simulink model "Practica_10_BER_PNRZ"  (R2020a)
settings: Solver=VariableStepAuto  StartTime=0.0  StopTime=StopTime  RelTol=1e-3
libraries: commutil2 x2, commchan3 x1, commrandsrc3 x1, commsink2 x1
settings Model: Creator=León Mora  LastModifiedBy=León Mora

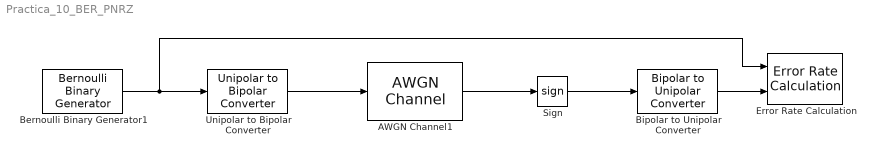
== system Practica_10_BER_PNRZ ==
  AWGN Channel1 : commchan3/AWGN Channel  InputProcessing=Columns as channels (frame based)  seed=67  noiseMode="Signal to noise ratio  (Eb/No)"  EbNodB=EbNo_k  EsNodB=10  SNRdB=10  bitsPerSym=1  Ps=1  Tsym=1  variance=1
  Bernoulli Binary Generator1 : commrandsrc3/Bernoulli Binary Generator  ProbabilityOfZero=0.5  SeedSource=Auto  Seed=0  SampleTime=1  SamplesPerFrame=FrameSize  OutputDataType=double  SimulateUsing=Interpreted execution
  Bipolar to Unipolar Converter : commutil2/Bipolar to Unipolar Converter  M=2  polarity=Positive  dataType=Inherit via internal rule
      settings: SourceProductBaseCode=CM
  Error Rate Calculation : commsink2/Error Rate Calculation  N=0  st_delay=0  cp_mode=Entire frame  subframe=[]  PMode=Workspace  WsName=ErrorVec  RsMode2=off  stop=off  numErr=100  maxBits=1e6
  Sign : Signum
  Unipolar to Bipolar Converter : commutil2/Unipolar to Bipolar Converter  M=2  polarity=Positive  dataType=Inherit via internal rule
  wires:
  Sign/1 -> Bipolar to Unipolar Converter/1
  Bernoulli Binary Generator1/1 -> Error Rate Calculation/1, Unipolar to Bipolar Converter/1
  Unipolar to Bipolar Converter/1 -> AWGN Channel1/1
  AWGN Channel1/1 -> Sign/1
  Bipolar to Unipolar Converter/1 -> Error Rate Calculation/2
